simulink model "LACS"  (R2016b)
settings: Solver=VariableStepAuto  StartTime=0.0  StopTime=10  RelTol=1e-3
values from neighbouring files (symbols this model uses):
  coefficient = 0.8    [LACS.sldd]
  Detal_ref = 0.00022116955850615819 0.00022116955850615819 0.00024339323736781077 0.00026784369743330114 0.00029474273075037104 0.00032433393975435165 0.00035688482250496254 0.00039268904453642435 0.00043206891122917146 0.00047537805500027884 0.00052300435183202216 0.00057537308165349073 0.00063295034678974044 0.00069624676200566427 0.00076582142849131239 0.0008422862023284908 0.000926310265386283 0.0010186250    [LACS.sldd]    (also in path_generate.m = zeros(N,1))
  driver_decel = 4.0    [LACS.sldd]
  EgoLength = 3.048    [LACS.sldd]
  egopath = 0.0 0.25 0.5 0.75 1.0 1.25 1.5 1.7500000000000002 2.0 2.25 2.5 2.75 3.0 3.25 3.5000000000000004 3.75 4.0 4.25 4.5 4.75 5.0 5.25 5.5 5.75 6.0 6.25 6.5 6.75 7.0000000000000009 7.2499999999999991 7.5 7.75 8.0 8.25 8.5 8.75 9.0 9.25 9.5 9.75 10.0 10.25 10.5 10.75 11.0 11.25 11.5 11.75 12.0 12.25 12.5 12.75 13.0 13.25 13.5 13.750000000000002 14.000000000000002 14.250000000000002 14.499999999999998 14.7    [LACS.sldd]
  egoSpdLimit_H = 150.0    [LACS.sldd]
  egoSpdLimit_L = 10.0    [LACS.sldd]
  EgoWidth = 1.628    [LACS.sldd]
  ESA_Active = 3.0    [LACS.sldd]
  ESA_mask_1 = 31.0    [LACS.sldd]
  ESA_mask_2 = 15.0    [LACS.sldd]
  ESA_mask_3 = 255.0    [LACS.sldd]
  ESA_mask_4 = 31.0    [LACS.sldd]
  ESA_Passive = 1.0    [LACS.sldd]
  ESA_Standby = 2.0    [LACS.sldd]
  g = 9.8    [LACS.sldd]
  headwayoffset = 1.524    [LACS.sldd]
  LatAccelThershold = 0.05    [LACS.sldd]
  LatDis = 0.5    [LACS.sldd]
  LatSafetyThershold = 0.5    [LACS.sldd]
  LengthObj = 3.0    [LACS.sldd]
  ObjWidth = 2.0    [LACS.sldd]
  PB1_decel = 3.0    [LACS.sldd]
  PB2_decel = 5.0    [LACS.sldd]
  PB3_decel = 8.0    [LACS.sldd]
  Phi_dot_ref = 0.00085065224568106894 0.00085065224568106894 0.000936127966106986 0.0010301682404378703 0.0011336261186052523 0.0012474385378394444 0.001372634343205976 0.0015103430260158721 0.001661804233646022 0.0018283781058153412 0.0020115564932359636 0.0022129751145658549 0.0024344267064660809 0.0026778752189651235 0.0029454711038487576 0.0032395677369184911 0.0035627390050890382 0.0039177980756855638 0.004    [LACS.sldd]    (also in path_generate.m = zeros(N,1))
  Phi_ref = 0.00038406250525431664 0.00042271073336932769 0.00046524334565338114 0.00051204974395873044 0.000563558155980624 0.00062023946191088657 0.00068261138880285879 0.00075124310596315759 0.0008267602572639512 0.0009098504689462523 0.0010012693742370194 0.0011018471988988175 0.0012124959546271103 0.0013342172899504143 0.0014681110508986705 0.0016153846060911084 0.0017773629929370329 0.001955499943191484    [LACS.sldd]    (also in path_generate.m = phi_ref)
  SteerAngleLimit = 20.0    [LACS.sldd]
  SteerAngleSpdLimit = 20.0    [LACS.sldd]
  StrAngSpdThershold = 0.05    [LACS.sldd]
  StrAngThershold = 0.0    [LACS.sldd]
  Time2React = 1.2    [LACS.sldd]
  timeMargin = 0.5    [LACS.sldd]
  TTCthreshold1 = 2.5    [LACS.sldd]
  TTCthreshold3 = 1.0    [LACS.sldd]
  X_dot_ref = 10.0 10.0 10.0 9.9999999999999947 10.0 10.0 10.0 10.0 10.0 10.0 10.0 10.0 10.0 10.0 10.0 10.000000000000018 10.0 10.0 10.0 10.0 10.0 10.0 10.0 10.0 10.0 10.0 10.0 10.0 10.0 10.0 10.0 10.0 10.0 10.0 10.0 10.0 10.0 10.0 10.0 10.0 10.0 10.0 10.0 10.0 10.0 10.0 10.0 10.0 10.0 10.0 10.0 10.0 10.0 10.0 10.0 10.0 10.0 10.0 10.0 10.0 10.0 10.0 10.0 9.9999999999999289 10.0 10.0 10.0 10.0 10.0 10.0 10.0 10.    [LACS.sldd]    (also in path_generate.m = zeros(N,1))
  X_ref = 0.05 0.55 1.05 1.55 2.05 2.55 3.05 3.55 4.05 4.55 5.05 5.55 6.05 6.55 7.05 7.55 8.05 8.55 9.05 9.55 10.05 10.55 11.05 11.55 12.05 12.55 13.05 13.55 14.05 14.55 15.05 15.55 16.05 16.55 17.05 17.55 18.05 18.55 19.05 19.55 20.05 20.55 21.05 21.55 22.05 22.55 23.05 23.55 24.05 24.55 25.05 25.55 26.05 26.55 27.05 27.55 28.05 28.55 29.05 29.55 30.05 30.55 31.05 31.55 32.05 32.55 33.05 33.55 34.05 34.55    [LACS.sldd]    (also in path_generate.m = X_phi')
  Y_dot_ref = 0.0044363771042237217 0.0044363771042237217 0.00488273213335339 0.0053739322979981 0.0059144698111347933 0.0065092840662692251 0.0071638055584438178 0.0078840039934084845 0.0086764409570179273 0.0095483275445279979 0.01050758737719603 0.011562925461771293 0.012723903376023141 0.014001021290828194 0.015405807364013962 0.016950915064438028 0.018650229002128878 0.020518979854070446 0.0225738689793052    [LACS.sldd]    (also in path_generate.m = zeros(N,1))
  Y_ref = 0.0020016327462461514 0.0022031718511841521 0.0024249907063953382 0.0026691273130630077 0.0029378239279629127 0.0032335474185196523 0.0035590116218331136 0.0039172018997553045 0.0043114020994257287 0.0047452241472766251 0.005222640524503025 0.0057480198933628265 0.0063261661664513911 0.0069623613352525482 0.0076624123997939579 0.008432702767994656 0.0092802485212165574 0.010212759971323001 0.01123    [LACS.sldd]    (also in path_generate.m = zeros(N,1))
undefined symbols (not defined in the file or in its folder): ADR_ADRCycleTime, ADR_SteeringYawrateThresh_p, AEB_mask1, aubr, CAEB_AccelPdlPosLimit, CAEB_AccelPdlPosSpdThreshold, CAEB_CalAEBLongVelObjLimit_mps, CAEB_CalAEBVMaxDec_kmph, ESA_AESACTIVE, ESA_ERROR, ESA_ESAFunctionOFF, ESA_ESAFunctionON, ESA_ESASwichOFF, ESA_ESS_DriverSteeringNumThreshold, ESA_ESSACTIVE, ESA_ForewardCollissionLevel2, ESA_ForewardCollissionLevel3, ESA_OFF, ESA_PASSIVE, ESA_PLAN_AES, ESA_PLAN_ESSLEFT, ESA_PLAN_ESSRIGHT, ESA_PLAN_FAILURE, ESA_PLAN_OFF, ESA_PLAN_STANDBY, ESA_PLAN_WAIT, ESA_SPEEDLIMITH6_p, ESA_SPEEDLIMITH7_p, ESA_SPEEDLIMITL6_p, ESA_SPEEDLIMITL7_p, ESA_STANDBY, ESA_StrAngSpdT6_p, FromAngle2Rad, Kp, magnitude, tablebr, TTCthreshold, vubr
libraries: simulink x15, Solver_SF x9, simulink_extras x1
(part 3 of 5)

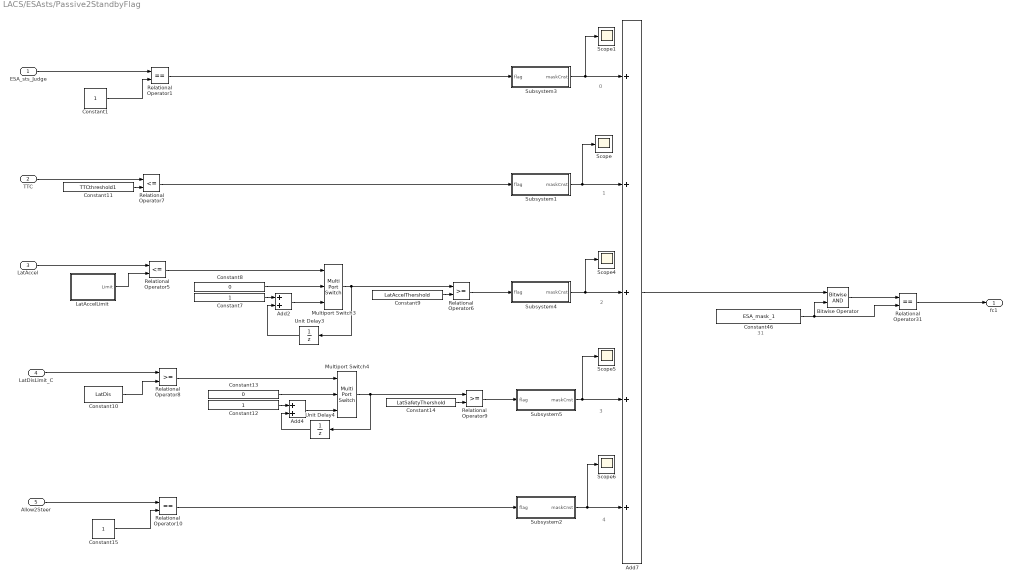
== system LACS/ESAsts/Passive2StandbyFlag ==
  note: 4
  note: 3
  note: 2
  note: 1
  note: 0
  note: 31
  ESA_sts_Judge : Inport
  TTC : Inport  Port=2
  LatAccel : Inport  Port=3
  LatDisLimit_C : Inport  Port=4
  Allow2Steer : Inport  Port=5
  Add2 : Sum  SaturateOnIntegerOverflow=on
  Add4 : Sum  SaturateOnIntegerOverflow=on
  Add7 : Sum  Inputs=5  SaturateOnIntegerOverflow=on
  Bitwise Operator : simulink/Logic and Bit Operations/Bitwise Operator  logicop=AND  UseBitMask=off  NumInputPorts=2  BitMask=bin2dec('11011001')  BitMaskRealWorld=Stored Integer
  Constant1 : Constant
  Constant10 : Constant  Value=LatDis
  Constant11 : Constant  Value=TTCthreshold1
  Constant12 : Constant  OutDataTypeStr=uint8
  Constant13 : Constant  Value=0  OutDataTypeStr=uint8
  Constant14 : Constant  Value=LatSafetyThershold
  Constant15 : Constant
  Constant46 : Constant  Value=ESA_mask_1  OutDataTypeStr=uint32
  Constant7 : Constant  OutDataTypeStr=uint8
  Constant8 : Constant  Value=0  OutDataTypeStr=uint8
  Constant9 : Constant  Value=LatAccelThershold
  LatAccelLimit : Subsystem
  Multiport Switch3 : MultiPortSwitch  DataPortOrder=Zero-based contiguous  Inputs=2
  Multiport Switch4 : MultiPortSwitch  DataPortOrder=Zero-based contiguous  Inputs=2
  Relational Operator1 : RelationalOperator  Operator===  OutDataTypeStr=boolean  RndMeth=Simplest
  Relational Operator10 : RelationalOperator  Operator===  OutDataTypeStr=boolean  RndMeth=Simplest
  Relational Operator31 : RelationalOperator  Operator===  OutDataTypeStr=boolean  RndMeth=Simplest
  Relational Operator5 : RelationalOperator  Operator=<=  OutDataTypeStr=boolean  RndMeth=Simplest
  Relational Operator6 : RelationalOperator  OutDataTypeStr=boolean  RndMeth=Simplest
  Relational Operator7 : RelationalOperator  Operator=<=  OutDataTypeStr=boolean  RndMeth=Simplest
  Relational Operator8 : RelationalOperator  OutDataTypeStr=boolean  RndMeth=Simplest
  Relational Operator9 : RelationalOperator  OutDataTypeStr=boolean  RndMeth=Simplest
  Scope{,1,4..6} (5 alike) : Scope
  Subsystem1 : Subsystem
  Subsystem2 : Subsystem
  Subsystem3 : Subsystem
  Subsystem4 : Subsystem
  Subsystem5 : Subsystem
  Unit Delay3 : UnitDelay  SampleTime=-1
  Unit Delay4 : UnitDelay  SampleTime=-1
  fc1 : Outport
  wires:
  Constant46/1 -> Bitwise Operator/2, Relational Operator31/2
  Bitwise Operator/1 -> Relational Operator31/1
  Relational Operator31/1 -> fc1/1
  Constant11/1 -> Relational Operator7/2
  TTC/1 -> Relational Operator7/1
  Relational Operator7/1 -> Subsystem1/1(flag)
  LatAccelLimit/1(Limit) -> Relational Operator5/2
  LatAccel/1 -> Relational Operator5/1
  Add2/1 -> Multiport Switch3/3
  Constant7/1 -> Add2/1
  Unit Delay3/1 -> Add2/2
  Constant8/1 -> Multiport Switch3/2
  Relational Operator5/1 -> Multiport Switch3/1
  Constant9/1 -> Relational Operator6/2
  Multiport Switch3/1 -> Unit Delay3/1, Relational Operator6/1
  Constant10/1 -> Relational Operator8/2
  LatDisLimit_C/1 -> Relational Operator8/1
  Add4/1 -> Multiport Switch4/3
  Constant12/1 -> Add4/1
  Unit Delay4/1 -> Add4/2
  Constant13/1 -> Multiport Switch4/2
  Relational Operator8/1 -> Multiport Switch4/1
  Constant14/1 -> Relational Operator9/2
  Multiport Switch4/1 -> Unit Delay4/1, Relational Operator9/1
  Relational Operator6/1 -> Subsystem4/1(flag)
  Relational Operator9/1 -> Subsystem5/1(flag)
  Subsystem1/1(maskCnst) -> Add7/2, Scope/1
  Subsystem4/1(maskCnst) -> Add7/3, Scope4/1
  Subsystem5/1(maskCnst) -> Add7/4, Scope5/1
  Add7/1 -> Bitwise Operator/1
  Constant15/1 -> Relational Operator10/2
  Allow2Steer/1 -> Relational Operator10/1
  Relational Operator10/1 -> Subsystem2/1(flag)
  Constant1/1 -> Relational Operator1/2
  ESA_sts_Judge/1 -> Relational Operator1/1
  Subsystem2/1(maskCnst) -> Add7/5, Scope6/1
  Relational Operator1/1 -> Subsystem3/1(flag)
  Subsystem3/1(maskCnst) -> Scope1/1, Add7/1

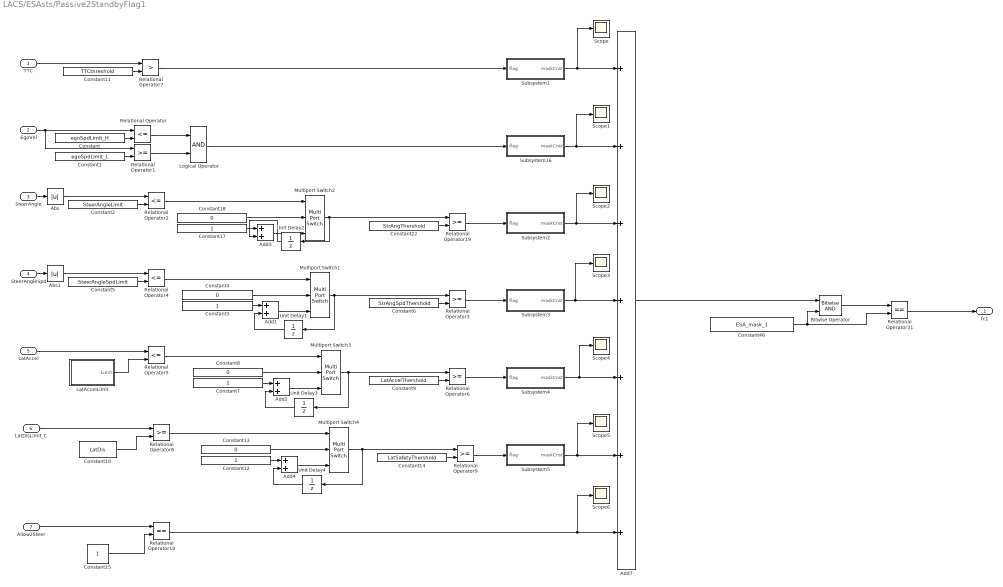
== system LACS/ESAsts/Passive2StandbyFlag1 ==
  TTC : Inport
  EgoVel : Inport  Port=2
  SteerAngle : Inport  Port=3
  SteerAngleSpd : Inport  Port=4
  LatAccel : Inport  Port=5
  LatDisLimit_C : Inport  Port=6
  Allow2Steer : Inport  Port=7
  Abs : Abs
  Abs1 : Abs
  Add{1..4} (4 alike) : Sum  SaturateOnIntegerOverflow=on
  Add7 : Sum  Inputs=7  SaturateOnIntegerOverflow=on
  Bitwise Operator : simulink/Logic and Bit Operations/Bitwise Operator  logicop=AND  UseBitMask=off  NumInputPorts=2  BitMask=bin2dec('11011001')  BitMaskRealWorld=Stored Integer
  Constant : Constant  Value=egoSpdLimit_H
  Constant1 : Constant  Value=egoSpdLimit_L
  Constant10 : Constant  Value=LatDis
  Constant11 : Constant  Value=TTCthreshold
  Constant{3,7,12,17} (4 alike) : Constant  OutDataTypeStr=uint8
  Constant{4,8,13,18} (4 alike) : Constant  Value=0  OutDataTypeStr=uint8
  Constant14 : Constant  Value=LatSafetyThershold
  Constant15 : Constant
  Constant2 : Constant  Value=SteerAngleLimit
  Constant22 : Constant  Value=StrAngThershold
  Constant46 : Constant  Value=ESA_mask_1  OutDataTypeStr=uint32
  Constant5 : Constant  Value=SteerAngleSpdLimit
  Constant6 : Constant  Value=StrAngSpdThershold
  Constant9 : Constant  Value=LatAccelThershold
  LatAccelLimit : Subsystem
  Logical Operator : Logic  AllPortsSameDT=off  OutDataTypeStr=boolean
  Multiport Switch{1..4} (4 alike) : MultiPortSwitch  DataPortOrder=Zero-based contiguous  Inputs=2
  Relational Operator{,2,4..5} (4 alike) : RelationalOperator  Operator=<=  OutDataTypeStr=boolean  RndMeth=Simplest
  Relational Operator{1,3,6,8..9,19} (6 alike) : RelationalOperator  OutDataTypeStr=boolean  RndMeth=Simplest
  Relational Operator10 : RelationalOperator  Operator===  OutDataTypeStr=boolean  RndMeth=Simplest
  Relational Operator31 : RelationalOperator  Operator===  OutDataTypeStr=boolean  RndMeth=Simplest
  Relational Operator7 : RelationalOperator  Operator=>  OutDataTypeStr=boolean  RndMeth=Simplest
  Scope{,1..6} (7 alike) : Scope
  Subsystem1 : Subsystem
  Subsystem16 : Subsystem
  Subsystem2 : Subsystem
  Subsystem3 : Subsystem
  Subsystem4 : Subsystem
  Subsystem5 : Subsystem
  Unit Delay{1..4} (4 alike) : UnitDelay  SampleTime=-1
  fc1 : Outport
  wires:
  Constant46/1 -> Bitwise Operator/2, Relational Operator31/2
  Bitwise Operator/1 -> Relational Operator31/1
  Relational Operator31/1 -> fc1/1
  Constant1/1 -> Relational Operator1/2
  Constant/1 -> Relational Operator/2
  EgoVel/1 -> Relational Operator/1, Relational Operator1/1
  Relational Operator1/1 -> Logical Operator/2
  Relational Operator/1 -> Logical Operator/1
  Logical Operator/1 -> Subsystem16/1(flag)
  Constant2/1 -> Relational Operator2/2
  SteerAngle/1 -> Abs/1
  Add3/1 -> Multiport Switch2/3
  Constant17/1 -> Add3/1
  Unit Delay2/1 -> Add3/2
  Constant22/1 -> Relational Operator19/2
  Multiport Switch2/1 -> Unit Delay2/1, Relational Operator19/1
  Constant18/1 -> Multiport Switch2/2
  Relational Operator2/1 -> Multiport Switch2/1
  Constant5/1 -> Relational Operator4/2
  SteerAngleSpd/1 -> Abs1/1
  Add1/1 -> Multiport Switch1/3
  Constant3/1 -> Add1/1
  Unit Delay1/1 -> Add1/2
  Constant6/1 -> Relational Operator3/2
  Multiport Switch1/1 -> Unit Delay1/1, Relational Operator3/1
  Constant4/1 -> Multiport Switch1/2
  Relational Operator4/1 -> Multiport Switch1/1
  Constant11/1 -> Relational Operator7/2
  TTC/1 -> Relational Operator7/1
  Relational Operator7/1 -> Subsystem1/1(flag)
  LatAccelLimit/1(Limit) -> Relational Operator5/2
  LatAccel/1 -> Relational Operator5/1
  Add2/1 -> Multiport Switch3/3
  Constant7/1 -> Add2/1
  Unit Delay3/1 -> Add2/2
  Constant8/1 -> Multiport Switch3/2
  Relational Operator5/1 -> Multiport Switch3/1
  Constant9/1 -> Relational Operator6/2
  Multiport Switch3/1 -> Unit Delay3/1, Relational Operator6/1
  Constant10/1 -> Relational Operator8/2
  LatDisLimit_C/1 -> Relational Operator8/1
  Add4/1 -> Multiport Switch4/3
  Constant12/1 -> Add4/1
  Unit Delay4/1 -> Add4/2
  Constant13/1 -> Multiport Switch4/2
  Relational Operator8/1 -> Multiport Switch4/1
  Constant14/1 -> Relational Operator9/2
  Multiport Switch4/1 -> Unit Delay4/1, Relational Operator9/1
  Relational Operator19/1 -> Subsystem2/1(flag)
  Relational Operator3/1 -> Subsystem3/1(flag)
  Relational Operator6/1 -> Subsystem4/1(flag)
  Relational Operator9/1 -> Subsystem5/1(flag)
  Subsystem1/1(maskCnst) -> Scope/1, Add7/1
  Subsystem16/1(maskCnst) -> Scope1/1, Add7/2
  Subsystem2/1(maskCnst) -> Scope2/1, Add7/3
  Subsystem3/1(maskCnst) -> Scope3/1, Add7/4
  Subsystem4/1(maskCnst) -> Scope4/1, Add7/5
  Subsystem5/1(maskCnst) -> Scope5/1, Add7/6
  Add7/1 -> Bitwise Operator/1
  Constant15/1 -> Relational Operator10/2
  Allow2Steer/1 -> Relational Operator10/1
  Relational Operator10/1 -> Scope6/1, Add7/7
  Abs/1 -> Relational Operator2/1
  Abs1/1 -> Relational Operator4/1

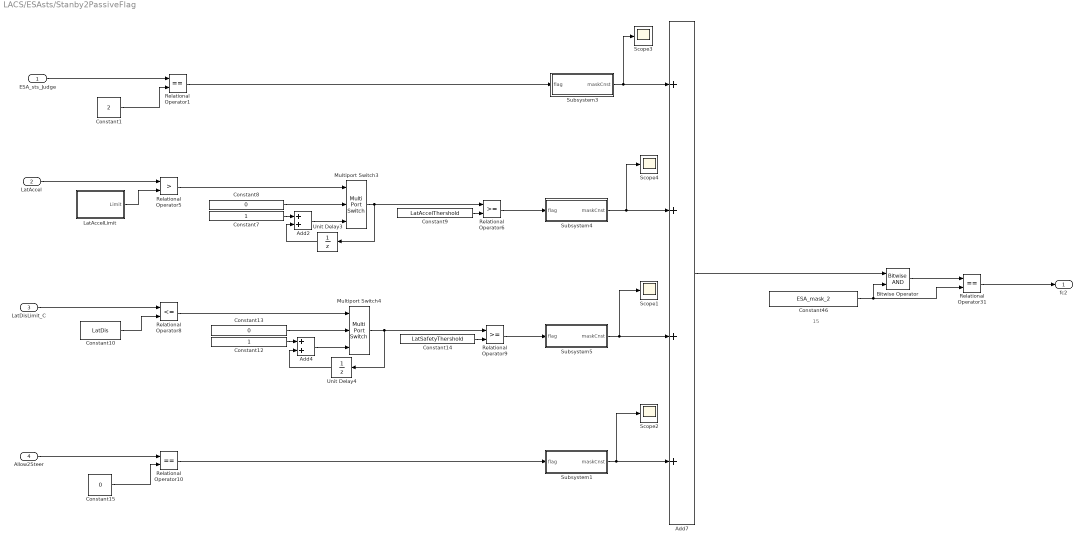
== system LACS/ESAsts/Stanby2PassiveFlag ==
  note: 15
  ESA_sts_Judge : Inport
  LatAccel : Inport  Port=2
  LatDisLimit_C : Inport  Port=3
  Allow2Steer : Inport  Port=4
  Add2 : Sum  SaturateOnIntegerOverflow=on
  Add4 : Sum  SaturateOnIntegerOverflow=on
  Add7 : Sum  Inputs=4  SaturateOnIntegerOverflow=on
  Bitwise Operator : simulink/Logic and Bit Operations/Bitwise Operator  logicop=AND  UseBitMask=off  NumInputPorts=2  BitMask=bin2dec('11011001')  BitMaskRealWorld=Stored Integer
  Constant1 : Constant  Value=2
  Constant10 : Constant  Value=LatDis
  Constant12 : Constant  OutDataTypeStr=uint8
  Constant13 : Constant  Value=0  OutDataTypeStr=uint8
  Constant14 : Constant  Value=LatSafetyThershold
  Constant15 : Constant  Value=0
  Constant46 : Constant  Value=ESA_mask_2  OutDataTypeStr=uint32
  Constant7 : Constant  OutDataTypeStr=uint8
  Constant8 : Constant  Value=0  OutDataTypeStr=uint8
  Constant9 : Constant  Value=LatAccelThershold
  LatAccelLimit : Subsystem
  Multiport Switch3 : MultiPortSwitch  DataPortOrder=Zero-based contiguous  Inputs=2
  Multiport Switch4 : MultiPortSwitch  DataPortOrder=Zero-based contiguous  Inputs=2
  Relational Operator1 : RelationalOperator  Operator===  OutDataTypeStr=boolean  RndMeth=Simplest
  Relational Operator10 : RelationalOperator  Operator===  OutDataTypeStr=boolean  RndMeth=Simplest
  Relational Operator31 : RelationalOperator  Operator===  OutDataTypeStr=boolean  RndMeth=Simplest
  Relational Operator5 : RelationalOperator  Operator=>  OutDataTypeStr=boolean  RndMeth=Simplest
  Relational Operator6 : RelationalOperator  OutDataTypeStr=boolean  RndMeth=Simplest
  Relational Operator8 : RelationalOperator  Operator=<=  OutDataTypeStr=boolean  RndMeth=Simplest
  Relational Operator9 : RelationalOperator  OutDataTypeStr=boolean  RndMeth=Simplest
  Scope{1..4} (4 alike) : Scope
  Subsystem1 : Subsystem
  Subsystem3 : Subsystem
  Subsystem4 : Subsystem
  Subsystem5 : Subsystem
  Unit Delay3 : UnitDelay  SampleTime=-1
  Unit Delay4 : UnitDelay  SampleTime=-1
  fc2 : Outport
  wires:
  Constant46/1 -> Bitwise Operator/2, Relational Operator31/2
  Bitwise Operator/1 -> Relational Operator31/1
  Relational Operator31/1 -> fc2/1
  LatAccelLimit/1(Limit) -> Relational Operator5/2
  LatAccel/1 -> Relational Operator5/1
  Add2/1 -> Multiport Switch3/3
  Constant7/1 -> Add2/1
  Unit Delay3/1 -> Add2/2
  Constant8/1 -> Multiport Switch3/2
  Relational Operator5/1 -> Multiport Switch3/1
  Constant9/1 -> Relational Operator6/2
  Multiport Switch3/1 -> Unit Delay3/1, Relational Operator6/1
  Constant10/1 -> Relational Operator8/2
  LatDisLimit_C/1 -> Relational Operator8/1
  Add4/1 -> Multiport Switch4/3
  Constant12/1 -> Add4/1
  Unit Delay4/1 -> Add4/2
  Constant13/1 -> Multiport Switch4/2
  Relational Operator8/1 -> Multiport Switch4/1
  Constant14/1 -> Relational Operator9/2
  Multiport Switch4/1 -> Unit Delay4/1, Relational Operator9/1
  Relational Operator6/1 -> Subsystem4/1(flag)
  Relational Operator9/1 -> Subsystem5/1(flag)
  Add7/1 -> Bitwise Operator/1
  Constant15/1 -> Relational Operator10/2
  Allow2Steer/1 -> Relational Operator10/1
  Subsystem4/1(maskCnst) -> Add7/2, Scope4/1
  Subsystem5/1(maskCnst) -> Scope1/1, Add7/3
  Relational Operator10/1 -> Subsystem1/1(flag)
  Constant1/1 -> Relational Operator1/2
  ESA_sts_Judge/1 -> Relational Operator1/1
  Relational Operator1/1 -> Subsystem3/1(flag)
  Subsystem3/1(maskCnst) -> Scope3/1, Add7/1
  Subsystem1/1(maskCnst) -> Add7/4, Scope2/1

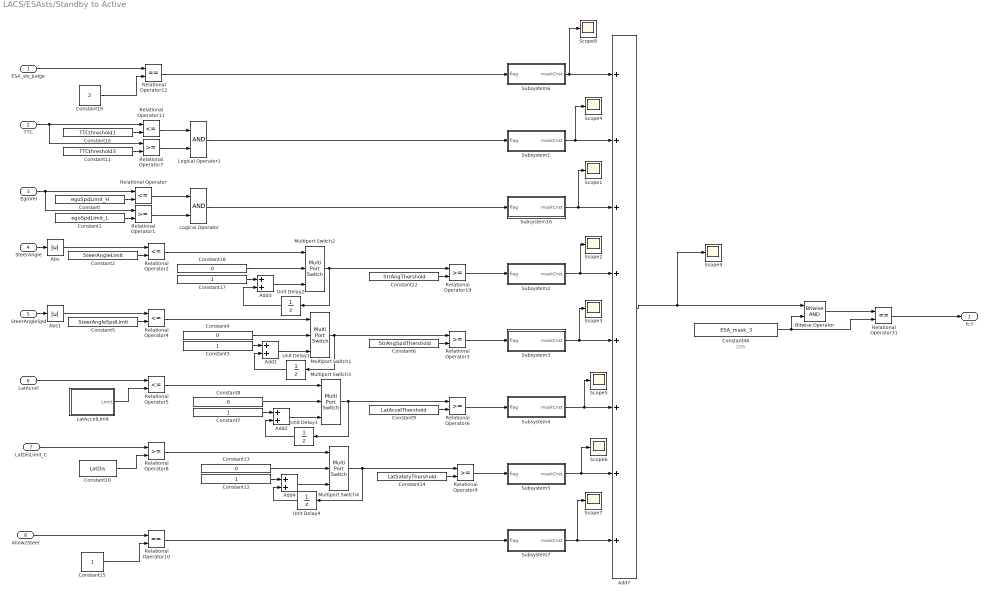
== system LACS/ESAsts/Standby to Active ==
  note: 255
  ESA_sts_Judge : Inport
  TTC : Inport  Port=2
  EgoVel : Inport  Port=3
  SteerAngle : Inport  Port=4
  SteerAngleSpd : Inport  Port=5
  LatAccel : Inport  Port=6
  LatDisLimit_C : Inport  Port=7
  Allow2Steer : Inport  Port=8
  Abs : Abs
  Abs1 : Abs
  Add{1..4} (4 alike) : Sum  SaturateOnIntegerOverflow=on
  Add7 : Sum  Inputs=8  SaturateOnIntegerOverflow=on
  Bitwise Operator : simulink/Logic and Bit Operations/Bitwise Operator  logicop=AND  UseBitMask=off  NumInputPorts=2  BitMask=bin2dec('11011001')  BitMaskRealWorld=Stored Integer
  Constant : Constant  Value=egoSpdLimit_H
  Constant1 : Constant  Value=egoSpdLimit_L
  Constant10 : Constant  Value=LatDis
  Constant11 : Constant  Value=TTCthreshold3
  Constant{3,7,12,17} (4 alike) : Constant  OutDataTypeStr=uint8
  Constant{4,8,13,18} (4 alike) : Constant  Value=0  OutDataTypeStr=uint8
  Constant14 : Constant  Value=LatSafetyThershold
  Constant15 : Constant
  Constant16 : Constant  Value=TTCthreshold1
  Constant19 : Constant  Value=2
  Constant2 : Constant  Value=SteerAngleLimit
  Constant22 : Constant  Value=StrAngThershold
  Constant46 : Constant  Value=ESA_mask_3  OutDataTypeStr=uint32
  Constant5 : Constant  Value=SteerAngleSpdLimit
  Constant6 : Constant  Value=StrAngSpdThershold
  Constant9 : Constant  Value=LatAccelThershold
  LatAccelLimit : Subsystem
  Logical Operator : Logic  AllPortsSameDT=off  OutDataTypeStr=boolean
  Logical Operator1 : Logic  AllPortsSameDT=off  OutDataTypeStr=boolean
  Multiport Switch{1..4} (4 alike) : MultiPortSwitch  DataPortOrder=Zero-based contiguous  Inputs=2
  Relational Operator{,2,4..5,11} (5 alike) : RelationalOperator  Operator=<=  OutDataTypeStr=boolean  RndMeth=Simplest
  Relational Operator{1,3,6..9,19} (7 alike) : RelationalOperator  OutDataTypeStr=boolean  RndMeth=Simplest
  Relational Operator10 : RelationalOperator  Operator===  OutDataTypeStr=boolean  RndMeth=Simplest
  Relational Operator12 : RelationalOperator  Operator===  OutDataTypeStr=boolean  RndMeth=Simplest
  Relational Operator31 : RelationalOperator  Operator===  OutDataTypeStr=boolean  RndMeth=Simplest
  Scope{1..9} (9 alike) : Scope
  Subsystem1 : Subsystem
  Subsystem16 : Subsystem
  Subsystem2 : Subsystem
  Subsystem3 : Subsystem
  Subsystem4 : Subsystem
  Subsystem5 : Subsystem
  Subsystem6 : Subsystem
  Subsystem7 : Subsystem
  Unit Delay{1..4} (4 alike) : UnitDelay  SampleTime=-1
  fc3 : Outport
  wires:
  Constant46/1 -> Bitwise Operator/2, Relational Operator31/2
  Bitwise Operator/1 -> Relational Operator31/1
  Relational Operator31/1 -> fc3/1
  Constant1/1 -> Relational Operator1/2
  Constant/1 -> Relational Operator/2
  EgoVel/1 -> Relational Operator/1, Relational Operator1/1
  Relational Operator1/1 -> Logical Operator/2
  Relational Operator/1 -> Logical Operator/1
  Logical Operator/1 -> Subsystem16/1(flag)
  Constant2/1 -> Relational Operator2/2
  SteerAngle/1 -> Abs/1
  Add3/1 -> Multiport Switch2/3
  Constant17/1 -> Add3/1
  Unit Delay2/1 -> Add3/2
  Constant22/1 -> Relational Operator19/2
  Multiport Switch2/1 -> Unit Delay2/1, Relational Operator19/1
  Constant18/1 -> Multiport Switch2/2
  Relational Operator2/1 -> Multiport Switch2/1
  Constant5/1 -> Relational Operator4/2
  SteerAngleSpd/1 -> Abs1/1
  Add1/1 -> Multiport Switch1/3
  Constant3/1 -> Add1/1
  Unit Delay1/1 -> Add1/2
  Constant6/1 -> Relational Operator3/2
  Multiport Switch1/1 -> Unit Delay1/1, Relational Operator3/1
  Constant4/1 -> Multiport Switch1/2
  Relational Operator4/1 -> Multiport Switch1/1
  Constant11/1 -> Relational Operator7/2
  LatAccelLimit/1(Limit) -> Relational Operator5/2
  LatAccel/1 -> Relational Operator5/1
  Add2/1 -> Multiport Switch3/3
  Constant7/1 -> Add2/1
  Unit Delay3/1 -> Add2/2
  Constant8/1 -> Multiport Switch3/2
  Relational Operator5/1 -> Multiport Switch3/1
  Constant9/1 -> Relational Operator6/2
  Multiport Switch3/1 -> Unit Delay3/1, Relational Operator6/1
  Constant10/1 -> Relational Operator8/2
  LatDisLimit_C/1 -> Relational Operator8/1
  Add4/1 -> Multiport Switch4/3
  Constant12/1 -> Add4/1
  Unit Delay4/1 -> Add4/2
  Constant13/1 -> Multiport Switch4/2
  Relational Operator8/1 -> Multiport Switch4/1
  Constant14/1 -> Relational Operator9/2
  Multiport Switch4/1 -> Unit Delay4/1, Relational Operator9/1
  Relational Operator19/1 -> Subsystem2/1(flag)
  Relational Operator3/1 -> Subsystem3/1(flag)
  Relational Operator6/1 -> Subsystem4/1(flag)
  Relational Operator9/1 -> Subsystem5/1(flag)
  Subsystem1/1(maskCnst) -> Add7/2, Scope4/1
  Subsystem16/1(maskCnst) -> Add7/3, Scope1/1
  Subsystem2/1(maskCnst) -> Add7/4, Scope2/1
  Subsystem3/1(maskCnst) -> Add7/5, Scope3/1
  Subsystem4/1(maskCnst) -> Add7/6, Scope5/1
  Subsystem5/1(maskCnst) -> Add7/7, Scope6/1
  Add7/1 -> Scope9/1, Bitwise Operator/1
  Relational Operator10/1 -> Subsystem7/1(flag)
  Constant15/1 -> Relational Operator10/2
  Allow2Steer/1 -> Relational Operator10/1
  Abs/1 -> Relational Operator2/1
  Abs1/1 -> Relational Operator4/1
  TTC/1 -> Relational Operator7/1, Relational Operator11/1
  Constant16/1 -> Relational Operator11/2
  Relational Operator11/1 -> Logical Operator1/1
  Relational Operator7/1 -> Logical Operator1/2
  Logical Operator1/1 -> Subsystem1/1(flag)
  Constant19/1 -> Relational Operator12/2
  ESA_sts_Judge/1 -> Relational Operator12/1
  Relational Operator12/1 -> Subsystem6/1(flag)
  Subsystem6/1(maskCnst) -> Add7/1, Scope8/1
  Subsystem7/1(maskCnst) -> Add7/8, Scope7/1

== system LACS/ESAsts/TTCCaculation1 ==
  LongiDis : Inport
  LongiVel : Inport  Port=2
  Abs : Abs
  Abs1 : Abs
  Add : Sum  Inputs=+-
  Constant : Constant  Value=headwayoffset
  Constant1 : Constant  Value=0.1
  Divide : Product  Inputs=*/
  Relational Operator4 : RelationalOperator  Operator=<  OutDataTypeStr=boolean  RndMeth=Simplest
  collision : Outport
  TTC : Outport  Port=2
  wires:
  Relational Operator4/1 -> collision/1
  Constant1/1 -> Relational Operator4/2
  Constant/1 -> Add/2
  Add/1 -> Divide/1, Relational Operator4/1
  LongiDis/1 -> Add/1
  Abs/1 -> Divide/2
  Divide/1 -> Abs1/1
  LongiVel/1 -> Abs/1
  Abs1/1 -> TTC/1

== system LACS/AEB/ConditionAdaptAEB/Subsystem16 ==
  flag : Inport
  Constant45 : Constant  Value=0  OutDataTypeStr=uint32
  Constant46 : Constant  OutDataTypeStr=uint32
  Multiport Switch7 : MultiPortSwitch  DataPortOrder=Zero-based contiguous  Inputs=2
  Shift Arithmetic : ArithShift  BitShiftNumberSource=Input port  BitShiftNumber=8  BitShiftDirection=Left
      settings: InputPortMap=u0,p1
  bitMask : Constant  Value=0  OutDataTypeStr=uint8
  maskCnst : Outport
  wires:
  flag/1 -> Multiport Switch7/1
  Multiport Switch7/1 -> maskCnst/1
  Constant46/1 -> Shift Arithmetic/1
  Constant45/1 -> Multiport Switch7/2
  Shift Arithmetic/1 -> Multiport Switch7/3
  bitMask/1 -> Shift Arithmetic/2

== system LACS/AEB//ESAModeSwitch/If Action Subsystem1/If Action Subsystem ==
  AEBTTCVaild : Inport
  AEBTTC : Inport  Port=2
  EgoSpd : Inport  Port=3
  Action Port : ActionPort
  Logical Operator1 : Logic  AllPortsSameDT=off  OutDataTypeStr=boolean
  Relational Operator1 : RelationalOperator  Operator=>  OutDataTypeStr=boolean  RndMeth=Simplest
  Relational Operator2 : RelationalOperator  Operator=>  OutDataTypeStr=boolean  RndMeth=Simplest
  Relational Operator22 : RelationalOperator  Operator===  OutDataTypeStr=boolean  RndMeth=Simplest
  TTC1 : Constant  OutDataTypeStr=boolean
  TTC2 : Constant  Value=4  OutDataTypeStr=boolean
  TTC3 : Constant  Value=0  OutDataTypeStr=boolean
  ESAVTakeOverReq : Outport
  AEBVCrashAvoid : Outport  Port=2
  wires:
  Logical Operator1/1 -> ESAVTakeOverReq/1
  AEBTTCVaild/1 -> Relational Operator22/1
  TTC1/1 -> Relational Operator22/2
  Relational Operator22/1 -> AEBVCrashAvoid/1
  AEBTTC/1 -> Relational Operator1/1
  TTC2/1 -> Relational Operator1/2
  Relational Operator1/1 -> Logical Operator1/1
  TTC3/1 -> Relational Operator2/2
  EgoSpd/1 -> Relational Operator2/1
  Relational Operator2/1 -> Logical Operator1/2

== system LACS/AEB//ESAModeSwitch/If Action Subsystem1/If Action Subsystem1 ==
  note: 60
  AEBTTC : Inport
  EgoSpd : Inport  Port=2
  Action Port : ActionPort
  CAEB_CalAEBVMaxDec_kmph : Constant  Value=CAEB_CalAEBVMaxDec_kmph
  Constant : Constant  Value=0  OutDataTypeStr=boolean
  Data Type Conversion : DataTypeConversion
  Data Type Conversion1 : DataTypeConversion
  Logical Operator : Logic  AllPortsSameDT=off  OutDataTypeStr=boolean
  Logical Operator1 : Logic  AllPortsSameDT=off  OutDataTypeStr=boolean
  Relational Operator : RelationalOperator  Operator=<=  OutDataTypeStr=boolean  RndMeth=Simplest
  Relational Operator1 : RelationalOperator  Operator===  OutDataTypeStr=boolean  RndMeth=Simplest
  Relational Operator2 : RelationalOperator  Operator=>  OutDataTypeStr=boolean  RndMeth=Simplest
  Relational Operator3 : RelationalOperator  Operator=>  OutDataTypeStr=boolean  RndMeth=Simplest
  TTC2 : Constant  Value=4  OutDataTypeStr=boolean
  TTC3 : Constant  Value=0  OutDataTypeStr=boolean
  ESAVTakeOverReq : Outport
  AEBVCrashAvoid : Outport  Port=2
  wires:
  Data Type Conversion1/1 -> ESAVTakeOverReq/1
  Data Type Conversion/1 -> AEBVCrashAvoid/1
  Relational Operator1/1 -> Logical Operator/1
  Constant/1 -> Relational Operator1/2
  Relational Operator/1 -> Data Type Conversion/1, Relational Operator1/1
  Logical Operator/1 -> Data Type Conversion1/1
  CAEB_CalAEBVMaxDec_kmph/1 -> Relational Operator/2
  AEBTTC/1 -> Relational Operator2/1
  TTC2/1 -> Relational Operator2/2
  Relational Operator2/1 -> Logical Operator1/1
  TTC3/1 -> Relational Operator3/2
  Relational Operator3/1 -> Logical Operator1/2
  Logical Operator1/1 -> Logical Operator/2
  EgoSpd/1 -> Relational Operator3/1, Relational Operator/1

== system LACS/AEB//ESAModeSwitch/If Action Subsystem1/If Action Subsystem2 ==
  Action Port : ActionPort
  Constant : Constant  Value=0  OutDataTypeStr=boolean
  Constant2 : Constant  OutDataTypeStr=boolean
  ESAVTakeOverReq : Outport
  AEBVCrashAvoid : Outport  Port=2
  wires:
  Constant/1 -> ESAVTakeOverReq/1
  Constant2/1 -> AEBVCrashAvoid/1

== system LACS/ESA/ConditionAdaptESA/Subsystem16 ==
  flag : Inport
  Constant45 : Constant  Value=0  OutDataTypeStr=uint32
  Constant46 : Constant  OutDataTypeStr=uint32
  Multiport Switch7 : MultiPortSwitch  DataPortOrder=Zero-based contiguous  Inputs=2
  Shift Arithmetic : ArithShift  BitShiftNumberSource=Input port  BitShiftNumber=8  BitShiftDirection=Left
      settings: InputPortMap=u0,p1
  bitMask : Constant  Value=0  OutDataTypeStr=uint8
  maskCnst : Outport
  wires:
  flag/1 -> Multiport Switch7/1
  Multiport Switch7/1 -> maskCnst/1
  Constant46/1 -> Shift Arithmetic/1
  Constant45/1 -> Multiport Switch7/2
  Shift Arithmetic/1 -> Multiport Switch7/3
  bitMask/1 -> Shift Arithmetic/2

== system LACS/ESA/SteerDirection/If Action Subsystem1 ==
  Action Port : ActionPort  ActionType=else
  Constant : Constant  Value=0
  Out1 : Outport
  wires:
  Constant/1 -> Out1/1

== system LACS/ESA/SteerDirection/Subsystem ==
  In1 : Inport
  Action Port : ActionPort  ActionType=then
  Add3 : Sum  SaturateOnIntegerOverflow=on
  Constant : Constant  Value=0
  Constant17 : Constant  OutDataTypeStr=uint8
  Constant18 : Constant  Value=0  OutDataTypeStr=uint8
  Constant22 : Constant  Value=ESA_ESS_DriverSteeringNumThreshold
  Delay : Delay  DelayLength=1  InitialCondition=0
  Divide : Product  Inputs=**
  Multiport Switch2 : MultiPortSwitch  DataPortOrder=Zero-based contiguous  Inputs=2
  Relational Operator : RelationalOperator  Operator=>  OutDataTypeStr=boolean  RndMeth=Simplest
  Relational Operator19 : RelationalOperator  OutDataTypeStr=boolean  RndMeth=Simplest
  Unit Delay2 : UnitDelay  SampleTime=-1
  Out2 : Outport
  wires:
  Relational Operator19/1 -> Out2/1
  Divide/1 -> Relational Operator/1
  Delay/1 -> Divide/2
  Constant/1 -> Relational Operator/2
  Multiport Switch2/1 -> Relational Operator19/1, Unit Delay2/1
  Constant22/1 -> Relational Operator19/2
  Add3/1 -> Multiport Switch2/3
  Constant17/1 -> Add3/1
  Unit Delay2/1 -> Add3/2
  Constant18/1 -> Multiport Switch2/2
  Relational Operator/1 -> Multiport Switch2/1
  In1/1 -> Delay/1, Divide/1

== system LACS/ESA/SteerDirection/Subsystem1 ==
  In1 : Inport
  Action Port : ActionPort  ActionType=elseif
  Constant2 : Constant  Value=0
  Constant3 : Constant  Value=0
  Relational Operator2 : RelationalOperator  Operator=>  OutDataTypeStr=boolean  RndMeth=Simplest
  Relational Operator3 : RelationalOperator  Operator=<  OutDataTypeStr=boolean  RndMeth=Simplest
  Left : Outport
  Right : Outport  Port=2
  wires:
  Constant3/1 -> Relational Operator3/2
  In1/1 -> Relational Operator2/1, Relational Operator3/1
  Relational Operator3/1 -> Left/1
  Constant2/1 -> Relational Operator2/2
  Relational Operator2/1 -> Right/1

== system LACS/ESA/TrajactoryPlan/Steering ==
  yawrate : Inport
  velocity : Inport  Port=2
  Add : Sum  Inputs=+-
  Bus Creator : BusCreator  Inputs=3  OutDataTypeStr=Bus: ADRPosition_struct  NonVirtualBus=on
  Constant : Constant  Value=ADR_ADRCycleTime  OutDataTypeStr=single
  Constant1 : Constant  OutDataTypeStr=single
  Data Type Conversion : DataTypeConversion  OutDataTypeStr=single
  Data Type Conversion1 : DataTypeConversion  OutDataTypeStr=single
  Data Type Conversion2 : DataTypeConversion  OutDataTypeStr=single
  Divide : Product  Inputs=*/
  Product : Product
  Product1 : Product
  Product2 : Product
  Trigonometric Function : Trigonometry
  Trigonometric Function1 : Trigonometry  Operator=cos
  dPos_ego : Outport  OutDataTypeStr=Bus: ADRPosition_struct
  wires:
  Bus Creator/1 -> dPos_ego/1
  Data Type Conversion2/1 -> Bus Creator/3  "theta"
  Data Type Conversion1/1 -> Bus Creator/2  "y"
  Data Type Conversion/1 -> Bus Creator/1  "x"
  Product2/1 -> Data Type Conversion1/1
  Add/1 -> Product2/2
  Constant1/1 -> Add/1
  Trigonometric Function1/1 -> Add/2
  Product1/1 -> Data Type Conversion/1
  Trigonometric Function/1 -> Product1/2
  Product/1 -> Trigonometric Function/1, Trigonometric Function1/1, Data Type Conversion2/1  "ADR_M_EgoTheta"
  Constant/1 -> Product/2
  Divide/1 -> Product2/1, Product1/1  "ADR_M_EgoTrajRadius"
  velocity/1 -> Divide/1
  yawrate/1 -> Divide/2, Product/1

== system LACS/ESA/TrajactoryPlan/Straight ==
  velocity : Inport
  Bus Creator : BusCreator  Inputs=3  OutDataTypeStr=Bus: ADRPosition_struct  NonVirtualBus=on
  Constant : Constant  Value=0  OutDataTypeStr=single
  Constant1 : Constant  Value=ADR_ADRCycleTime  OutDataTypeStr=single
  Constant2 : Constant  Value=0  OutDataTypeStr=single
  Data Type Conversion : DataTypeConversion  OutDataTypeStr=single
  Data Type Conversion1 : DataTypeConversion  OutDataTypeStr=single
  Data Type Conversion2 : DataTypeConversion  OutDataTypeStr=single
  Product : Product
  dPos_ego : Outport  OutDataTypeStr=Bus: ADRPosition_struct
  wires:
  Bus Creator/1 -> dPos_ego/1
  Data Type Conversion2/1 -> Bus Creator/3  "theta"
  Data Type Conversion1/1 -> Bus Creator/2  "y"
  Data Type Conversion/1 -> Bus Creator/1  "x"
  Constant2/1 -> Data Type Conversion2/1
  Constant1/1 -> Product/2
  velocity/1 -> Product/1
  Product/1 -> Data Type Conversion/1
  Constant/1 -> Data Type Conversion1/1

== system LACS/ESAsts/Active to Passive/LatAccelLimit ==
  Constant10 : Constant  Value=g
  Constant12 : Constant  Value=0.67
  Constant9 : Constant  Value=coefficient
  Divide : Product  Inputs=***
  Limit : Outport
  wires:
  Constant10/1 -> Divide/2
  Constant12/1 -> Divide/3
  Divide/1 -> Limit/1
  Constant9/1 -> Divide/1

== system LACS/ESAsts/Active to Passive/Subsystem1 ==
  flag : Inport
  Constant45 : Constant  Value=0  OutDataTypeStr=uint32
  Constant46 : Constant  OutDataTypeStr=uint32
  Multiport Switch7 : MultiPortSwitch  DataPortOrder=Zero-based contiguous  Inputs=2
  Shift Arithmetic : ArithShift  BitShiftNumberSource=Input port  BitShiftNumber=8  BitShiftDirection=Left
      settings: InputPortMap=u0,p1
  bitMask : Constant  OutDataTypeStr=uint8
  maskCnst : Outport
  wires:
  flag/1 -> Multiport Switch7/1
  Multiport Switch7/1 -> maskCnst/1
  Constant46/1 -> Shift Arithmetic/1
  Constant45/1 -> Multiport Switch7/2
  Shift Arithmetic/1 -> Multiport Switch7/3
  bitMask/1 -> Shift Arithmetic/2

== system LACS/ESAsts/Active to Passive/Subsystem16 ==
  flag : Inport
  Constant45 : Constant  Value=0  OutDataTypeStr=uint32
  Constant46 : Constant  OutDataTypeStr=uint32
  Multiport Switch7 : MultiPortSwitch  DataPortOrder=Zero-based contiguous  Inputs=2
  Shift Arithmetic : ArithShift  BitShiftNumberSource=Input port  BitShiftNumber=8  BitShiftDirection=Left
      settings: InputPortMap=u0,p1
  bitMask : Constant  Value=2  OutDataTypeStr=uint8
  maskCnst : Outport
  wires:
  flag/1 -> Multiport Switch7/1
  Multiport Switch7/1 -> maskCnst/1
  Constant46/1 -> Shift Arithmetic/1
  Constant45/1 -> Multiport Switch7/2
  Shift Arithmetic/1 -> Multiport Switch7/3
  bitMask/1 -> Shift Arithmetic/2

== system LACS/ESAsts/Active to Passive/Subsystem2 ==
  flag : Inport
  Constant45 : Constant  Value=0  OutDataTypeStr=uint32
  Constant46 : Constant  OutDataTypeStr=uint32
  Multiport Switch7 : MultiPortSwitch  DataPortOrder=Zero-based contiguous  Inputs=2
  Shift Arithmetic : ArithShift  BitShiftNumberSource=Input port  BitShiftNumber=8  BitShiftDirection=Left
      settings: InputPortMap=u0,p1
  bitMask : Constant  Value=3  OutDataTypeStr=uint8
  maskCnst : Outport
  wires:
  bitMask/1 -> Shift Arithmetic/2
  Shift Arithmetic/1 -> Multiport Switch7/3
  Constant45/1 -> Multiport Switch7/2
  Constant46/1 -> Shift Arithmetic/1
  Multiport Switch7/1 -> maskCnst/1
  flag/1 -> Multiport Switch7/1

== system LACS/ESAsts/Active to Passive/Subsystem4 ==
  flag : Inport
  Constant45 : Constant  Value=0  OutDataTypeStr=uint32
  Constant46 : Constant  OutDataTypeStr=uint32
  Multiport Switch7 : MultiPortSwitch  DataPortOrder=Zero-based contiguous  Inputs=2
  Shift Arithmetic : ArithShift  BitShiftNumberSource=Input port  BitShiftNumber=8  BitShiftDirection=Left
      settings: InputPortMap=u0,p1
  bitMask : Constant  Value=4  OutDataTypeStr=uint8
  maskCnst : Outport
  wires:
  flag/1 -> Multiport Switch7/1
  Multiport Switch7/1 -> maskCnst/1
  Constant46/1 -> Shift Arithmetic/1
  Constant45/1 -> Multiport Switch7/2
  Shift Arithmetic/1 -> Multiport Switch7/3
  bitMask/1 -> Shift Arithmetic/2

== system LACS/ESAsts/Active to Passive/Subsystem5 ==
  flag : Inport
  Constant45 : Constant  Value=0  OutDataTypeStr=uint32
  Constant46 : Constant  OutDataTypeStr=uint32
  Multiport Switch7 : MultiPortSwitch  DataPortOrder=Zero-based contiguous  Inputs=2
  Shift Arithmetic : ArithShift  BitShiftNumberSource=Input port  BitShiftNumber=8  BitShiftDirection=Left
      settings: InputPortMap=u0,p1
  bitMask : Constant  Value=5  OutDataTypeStr=uint8
  maskCnst : Outport
  wires:
  flag/1 -> Multiport Switch7/1
  Multiport Switch7/1 -> maskCnst/1
  Constant46/1 -> Shift Arithmetic/1
  Constant45/1 -> Multiport Switch7/2
  Shift Arithmetic/1 -> Multiport Switch7/3
  bitMask/1 -> Shift Arithmetic/2

== system LACS/ESAsts/Active to Passive/Subsystem6 ==
  flag : Inport
  Constant45 : Constant  Value=0  OutDataTypeStr=uint32
  Constant46 : Constant  OutDataTypeStr=uint32
  Multiport Switch7 : MultiPortSwitch  DataPortOrder=Zero-based contiguous  Inputs=2
  Shift Arithmetic : ArithShift  BitShiftNumberSource=Input port  BitShiftNumber=8  BitShiftDirection=Left
      settings: InputPortMap=u0,p1
  bitMask : Constant  Value=0  OutDataTypeStr=uint8
  maskCnst : Outport
  wires:
  flag/1 -> Multiport Switch7/1
  Multiport Switch7/1 -> maskCnst/1
  Constant46/1 -> Shift Arithmetic/1
  Constant45/1 -> Multiport Switch7/2
  Shift Arithmetic/1 -> Multiport Switch7/3
  bitMask/1 -> Shift Arithmetic/2

== system LACS/ESAsts/LatDisSafetyLimit1/Dis4MassPoint2RightAngle ==
  Add : Sum
  Constant1 : Constant  Value=EgoWidth
  Constant2 : Constant  Value=EgoLength
  Gain : Gain  Gain=0.5
  Gain1 : Gain  Gain=0.5
  Math Function : Math  Operator=magnitude^2  SaturateOnIntegerOverflow=on
  Math Function1 : Math  Operator=magnitude^2  SaturateOnIntegerOverflow=on
  Sqrt : Sqrt  SaturateOnIntegerOverflow=on
  r1 : Outport
  wires:
  Constant1/1 -> Gain1/1
  Constant2/1 -> Gain/1
  Gain1/1 -> Math Function/1
  Gain/1 -> Math Function1/1
  Math Function/1 -> Add/1
  Math Function1/1 -> Add/2
  Add/1 -> Sqrt/1
  Sqrt/1 -> r1/1

== system LACS/ESAsts/Passive2StandbyFlag/LatAccelLimit ==
  Constant10 : Constant  Value=g
  Constant12 : Constant  Value=0.67
  Constant9 : Constant  Value=coefficient
  Divide : Product  Inputs=***
  Limit : Outport
  wires:
  Constant10/1 -> Divide/2
  Constant12/1 -> Divide/3
  Divide/1 -> Limit/1
  Constant9/1 -> Divide/1

== system LACS/ESAsts/Passive2StandbyFlag/Subsystem1 ==
  flag : Inport
  Constant45 : Constant  Value=0  OutDataTypeStr=uint32
  Constant46 : Constant  OutDataTypeStr=uint32
  Multiport Switch7 : MultiPortSwitch  DataPortOrder=Zero-based contiguous  Inputs=2
  Shift Arithmetic : ArithShift  BitShiftNumberSource=Input port  BitShiftNumber=8  BitShiftDirection=Left
      settings: InputPortMap=u0,p1
  bitMask : Constant  OutDataTypeStr=uint8
  maskCnst : Outport
  wires:
  flag/1 -> Multiport Switch7/1
  Multiport Switch7/1 -> maskCnst/1
  Constant46/1 -> Shift Arithmetic/1
  Constant45/1 -> Multiport Switch7/2
  Shift Arithmetic/1 -> Multiport Switch7/3
  bitMask/1 -> Shift Arithmetic/2

== system LACS/ESAsts/Passive2StandbyFlag/Subsystem2 ==
  flag : Inport
  Constant45 : Constant  Value=0  OutDataTypeStr=uint32
  Constant46 : Constant  OutDataTypeStr=uint32
  Multiport Switch7 : MultiPortSwitch  DataPortOrder=Zero-based contiguous  Inputs=2
  Shift Arithmetic : ArithShift  BitShiftNumberSource=Input port  BitShiftNumber=8  BitShiftDirection=Left
      settings: InputPortMap=u0,p1
  bitMask : Constant  Value=4  OutDataTypeStr=uint8
  maskCnst : Outport
  wires:
  flag/1 -> Multiport Switch7/1
  Multiport Switch7/1 -> maskCnst/1
  Constant46/1 -> Shift Arithmetic/1
  Constant45/1 -> Multiport Switch7/2
  Shift Arithmetic/1 -> Multiport Switch7/3
  bitMask/1 -> Shift Arithmetic/2
